simulink model "e8_4_FLY"  (R2017b)
settings: Solver=FixedStepDiscrete  StartTime=0.0  StopTime=10.0  RelTol=1e-3
values from neighbouring files (symbols this model uses):
  DEG2RAD = 0.0174533    [Init_control.m]
  Kd_PITCH_AngleRate = 0.001    [Init_control.m]
  Kd_ROLL_AngleRate = 0.001    [Init_control.m]
  Kd_YAW_AngleRate = 0.00    (= 0)    [Init_control.m]
  Ki_PITCH_AngleRate = 0.02    [Init_control.m]
  Ki_ROLL_AngleRate = 0.02    [Init_control.m]
  Ki_YAW_AngleRate = 0.01    [Init_control.m]
  Kp_PITCH_ANGLE = 6.5    [Init_control.m]
  Kp_PITCH_AngleRate = 0.1    [Init_control.m]
  Kp_ROLL_ANGLE = 6.5    [Init_control.m]
  Kp_ROLL_AngleRate = 0.1    [Init_control.m]
  Kp_YAW_ANGLE = 3    [Init_control.m]
  Kp_YAW_AngleRate = 0.5    [Init_control.m]
  Kpxp = 1.0    (= 1)    [Init_control.m]
  Kpyp = 1.0    (= 1)    [Init_control.m]
  Kpzp = 4.0    (= 4)    [Init_control.m]
  Kvxd = 0.01    [Init_control.m]
  Kvxi = 0.1    [Init_control.m]
  Kvxp = 3.0    (= 3)    [Init_control.m]
  Kvyd = 0.01    [Init_control.m]
  Kvyi = 0.1    [Init_control.m]
  Kvyp = 3.0    (= 3)    [Init_control.m]
  Kvzd = 0.005    [Init_control.m]
  Kvzi = 0.01    [Init_control.m]
  Kvzp = 0.45    [Init_control.m]
  MAX_CONTROL_ANGLE_NAV_PITCH = 15    [Init_control.m]
  MAX_CONTROL_ANGLE_NAV_ROLL = 15    [Init_control.m]
  MAX_CONTROL_ANGLE_PITCH = 35    [Init_control.m]
  MAX_CONTROL_ANGLE_RATE_PITCH = 220    [Init_control.m]
  MAX_CONTROL_ANGLE_RATE_ROLL = 220    [Init_control.m]
  MAX_CONTROL_ANGLE_RATE_Y = 200    [Init_control.m]
  MAX_CONTROL_ANGLE_ROLL = 35    [Init_control.m]
  MAX_CONTROL_VELOCITY_XY = 0.5    [Init_control.m]
  MAX_CONTROL_VELOCITY_Z = 1    [Init_control.m]
  Saturation_I_ah = 3.43    [Init_control.m]
  Saturation_I_az = 5    [Init_control.m]
  Saturation_I_RP_Max = 0.3    [Init_control.m]
  Saturation_I_RP_Min = -0.3    [Init_control.m]
  Saturation_I_Y_Max = 0.2    [Init_control.m]
  Saturation_I_Y_Min = -0.2    [Init_control.m]
  THR_HOVER = 0.609    [Init_control.m]
undefined symbols (not defined in the file or in its folder): DiscIntNeverNeededParam, KiRollAttitude, RGBLED_COLOR_ENUM, RGBLED_MODE_ENUM
libraries: simulink x12, pixhawk_slib_sensors_actuators x5, pixhawk_slib_uORB_RW x2
(part 2 of 2)

== matlab function e8_4_FLY/Control System/MATLAB Function2 ==
  data: ch5 input; MIE2_ output
function MIE2_ = fcn(ch5)
%Function description:
%  Map the remote CH5 channel to manual operation instructions
%Input:
%  ch5: Remote control CH5 channel input
%Output:
%  MIE2_:Manual operation instruction
%  1: MANUAL FLIGHT MODE
%  2: RTL MODE
%  3: AUTO-LANDING MODE
persistent mode1_count;
if isempty(mode1_count)
    mode1_count = 0;
end
persistent MIE2;
if isempty(MIE2)
    MIE2 = int8(0);
end

if ch5 < 1400
    MIE2 = int8(1);
    mode1_count = 0;
elseif ch5 < 1600
    mode1_count = mode1_count + 1;
    if mode1_count >= 100 % Anti-shake
        MIE2 = int8(2);
        if mode1_count > 1000
            mode1_count = 1000;
        end
    end
else
    MIE2 = int8(3);
    mode1_count = 0;
end

MIE2_ = MIE2;

== matlab function e8_4_FLY/Control System/MATLAB Function1 ==
  settings: updateMethod=DISCRETE
  data: state input; vxd output; vyd output; vzd output; x input; y input; z input; vx input; vy input; vz input; xd output; yd output; zd output
function [vxd, vyd, vzd, xd, yd, zd] = fcn(state, x, y, z, vx, vy, vz)
%Function description:
%  Flight mode switch  implemention.
%Input:
%  state: flight mode
%  x, y, z: current position
%  vx, vy,vz: current velocity
%Output:
%  vx_d, vy_d, vz_d: desired velocity
%  x_d, y_d, z_d: desired position
persistent hold_x_flag;
if isempty(hold_x_flag)
    hold_x_flag = 0;
end
persistent hold_y_flag;
if isempty(hold_y_flag)
    hold_y_flag = 0;
end
persistent hold_z_flag;
if isempty(hold_z_flag)
    hold_z_flag = 0;
end
persistent x1;
if isempty(x1)
    x1 = 0;
end
persistent y1;
if isempty(y1)
    y1 = 0;
end

persistent z1;
if isempty(z1)
    z1 = 0;
end

heightSafe = 5;  % desired height is set to 5 m
if state == 1  %Return, the altitude below the specified threshold, first rise to the specified value
    vxd = 0;  %Reduce the horizontal speed to 0
    vyd = 0;
    hold_x_flag = 0;
    hold_y_flag = 0;
    if abs(z) < heightSafe
        z1 = -heightSafe; vzd = 0; 
        hold_z_flag = 0;
    else
        vzd = 0;
        if abs(vz) < 6 &&(hold_z_flag < 0.5)
            z1 = z; 
            hold_z_flag = 1;
        end
        if ~(abs(vz) < 6)
           z1 = z;
           hold_z_flag = 0;
        end
    end
    
    if abs(vx) < 8
       x1 = 0; 
   end
   if ~(abs(vx) < 8)
       x1 = x; 
   end
   if abs(vy) < 8 
       y1 = 0;
   end
   if ~(abs(vy) < 8)
       y1 = y;
   end
elseif state == 2  %land
    vxd = 0; vyd = 0;
   z1 = 0; vzd = 0;  %desired height is 0,land
   hold_z_flag = 0;
   %olve the drift problem
   if abs(vx) < 8 && (hold_x_flag < 0.5)
       x1 = x; 
       hold_x_flag = 1;
   end
   if ~(abs(vx) < 8)
       x1 = x; 
       hold_x_flag = 0;
   end
   if abs(vy) < 8 && (hold_y_flag < 0.5)
       y1 = y;
       hold_y_flag = 1;
   end
   if ~(abs(vy) < 8)
       y1 = y;
       hold_y_flag = 0;
   end
   
else %mannual control mode
   x1 = x; vxd = 0;
   y1 = y; vyd = 0;
   z1 = z; vzd = 0;
   
   hold_x_flag = 0;
   hold_y_flag = 0;
   hold_z_flag = 0;
end

 xd = x1;
 yd = y1;
 zd = z1;
